simulink model "pendulum_PID"  (R2016a)
settings: Solver=VariableStepAuto  StartTime=0.0  StopTime=50  RelTol=1e-6
values from neighbouring files (symbols this model uses):
  A = [0 1 0 0 ... (first row only)    [main.m]
  B = [0; 1/M; 0; -1/(M*l)]    [main.m]
  C = [1 0 0 0 ... (first row only)    [main.m]
  D = [0; 0; 0; 0]    [main.m]
  K = dlqr(Ad,Bd,Q,R)    [main.m]
  Lwd = Ld(3,:)    [main.m]
  state0 = [x0, dx0, theta0, dtheta0]    [main.m]
undefined symbols (not defined in the file or in its folder): Ad, Bd, Cd, Dd, Den_d, L_db, M_db, Md, Num_d
libraries: simulink x11, fuzblock x2
settings Model: Creator=Maciej  LastModifiedBy=Maciej

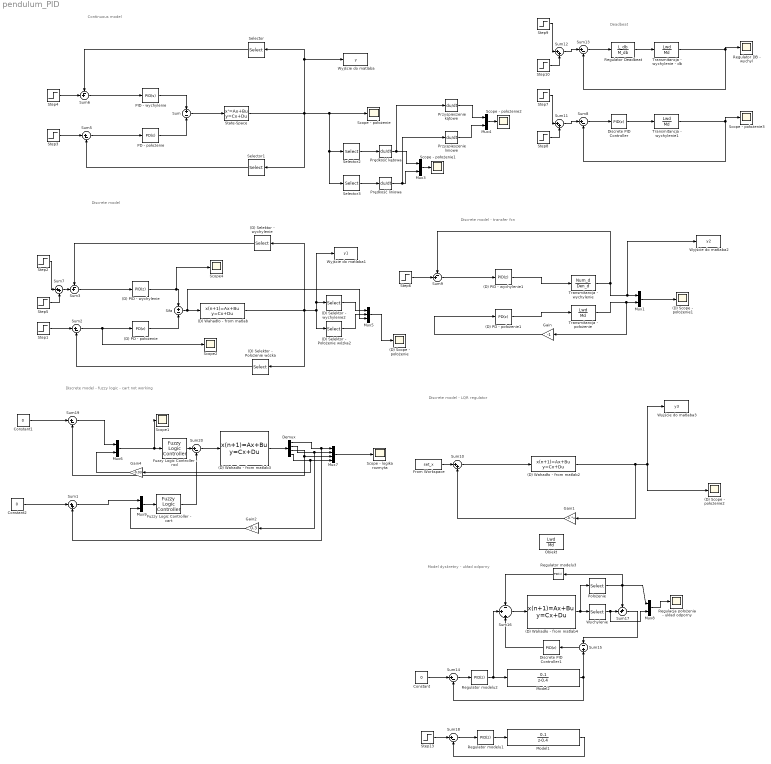
== system pendulum_PID ==
  note: Model dyskretny - układ odporny
  note: Deadbeat
  note: Discrete model - transfer fcn
  note: Discrete model - LQR regulator
  note: Discrete model
  note: Continuous model
  note: Discrete model - fuzzy logic - cart not working
  (D) PD - położenie : simulink/Continuous/PID Controller  Controller=PD  TimeDomain=Discrete-time  SampleTime=0.01  IntegratorMethod=Forward Euler  FilterMethod=Forward Euler  Form=Ideal  UseFilter=off  ControllerParametersSource=internal  P=12.6642993740103  I=0.264679114178146  D=0.005  N=100  InitialConditionSource=internal  InitialConditionForIntegrator=0  InitialConditionForFilter=0  ExternalReset=none  LimitOutput=off  UpperSaturationLimit=inf  LowerSaturationLimit=-inf  LinearizeAsGain=on  AntiWindupMode=none  Kb=1  TrackingMode=off  Kt=1  PParamMin=[]  PParamMax=[]  IParamMin=[]  IParamMax=[]  DParamMin=[]  DParamMax=[]  NParamMin=[]  NParamMax=[]  KbParamMin=[]  KbParamMax=[]  KtParamMin=[]  KtParamMax=[]  POutMin=[]  POutMax=[]  IOutMin=[]  IOutMax=[]  DOutMin=[]  DOutMax=[]  NOutMin=[]  NOutMax=[]  KbOutMin=[]  KbOutMax=[]  KtOutMin=[]  KtOutMax=[]  IntegratorOutMin=[]  IntegratorOutMax=[]  FilterOutMin=[]  FilterOutMax=[]  SumOutMin=[]  SumOutMax=[]  SumI1OutMin=[]  SumI1OutMax=[]  SumI2OutMin=[]  SumI2OutMax=[]  SumI3OutMin=[]  SumI3OutMax=[]  SumDOutMin=[]  SumDOutMax=[]  SaturationOutMin=[]  SaturationOutMax=[]  IntegratorContinuousStateAttributes=''  IntegratorStateMustResolveToSignalObject=off  IntegratorRTWStateStorageClass=Auto  FilterContinuousStateAttributes=''  FilterStateMustResolveToSignalObject=off  FilterRTWStateStorageClass=Auto  DifferentiatorICPrevScaledInput=0  DifferentiatorOutMin=[]  DifferentiatorOutMax=[]
  (D) PD - położenie1 : simulink/Continuous/PID Controller  Controller=PD  TimeDomain=Discrete-time  SampleTime=0.01  IntegratorMethod=Forward Euler  FilterMethod=Trapezoidal  Form=Ideal  UseFilter=on  ControllerParametersSource=internal  P=12.6641410705961  I=0.302421599344656  D=0  N=100  InitialConditionSource=internal  InitialConditionForIntegrator=0  InitialConditionForFilter=0  ExternalReset=none  LimitOutput=off  UpperSaturationLimit=inf  LowerSaturationLimit=-inf  LinearizeAsGain=on  AntiWindupMode=none  Kb=1  TrackingMode=off  Kt=1  PParamMin=[]  PParamMax=[]  IParamMin=[]  IParamMax=[]  DParamMin=[]  DParamMax=[]  NParamMin=[]  NParamMax=[]  KbParamMin=[]  KbParamMax=[]  KtParamMin=[]  KtParamMax=[]  POutMin=[]  POutMax=[]  IOutMin=[]  IOutMax=[]  DOutMin=[]  DOutMax=[]  NOutMin=[]  NOutMax=[]  KbOutMin=[]  KbOutMax=[]  KtOutMin=[]  KtOutMax=[]  IntegratorOutMin=[]  IntegratorOutMax=[]  FilterOutMin=[]  FilterOutMax=[]  SumOutMin=[]  SumOutMax=[]  SumI1OutMin=[]  SumI1OutMax=[]  SumI2OutMin=[]  SumI2OutMax=[]  SumI3OutMin=[]  SumI3OutMax=[]  SumDOutMin=[]  SumDOutMax=[]  SaturationOutMin=[]  SaturationOutMax=[]  IntegratorContinuousStateAttributes=''  IntegratorStateMustResolveToSignalObject=off  IntegratorRTWStateStorageClass=Auto  FilterContinuousStateAttributes=''  FilterStateMustResolveToSignalObject=off  FilterRTWStateStorageClass=Auto  DifferentiatorICPrevScaledInput=0  DifferentiatorOutMin=[]  DifferentiatorOutMax=[]
  (D) PID - wychylenie : simulink/Continuous/PID Controller  Controller=PID  TimeDomain=Discrete-time  SampleTime=0.01  IntegratorMethod=Forward Euler  FilterMethod=Forward Euler  Form=Ideal  UseFilter=on  ControllerParametersSource=internal  P=-46.8558412524277  I=2.71021165385829  D=0.0890699619507767  N=156.758466308077  InitialConditionSource=internal  InitialConditionForIntegrator=0  InitialConditionForFilter=0  ExternalReset=none  LimitOutput=off  UpperSaturationLimit=inf  LowerSaturationLimit=-inf  LinearizeAsGain=on  AntiWindupMode=none  Kb=1  TrackingMode=off  Kt=1  PParamMin=[]  PParamMax=[]  IParamMin=[]  IParamMax=[]  DParamMin=[]  DParamMax=[]  NParamMin=[]  NParamMax=[]  KbParamMin=[]  KbParamMax=[]  KtParamMin=[]  KtParamMax=[]  POutMin=[]  POutMax=[]  IOutMin=[]  IOutMax=[]  DOutMin=[]  DOutMax=[]  NOutMin=[]  NOutMax=[]  KbOutMin=[]  KbOutMax=[]  KtOutMin=[]  KtOutMax=[]  IntegratorOutMin=[]  IntegratorOutMax=[]  FilterOutMin=[]  FilterOutMax=[]  SumOutMin=[]  SumOutMax=[]  SumI1OutMin=[]  SumI1OutMax=[]  SumI2OutMin=[]  SumI2OutMax=[]  SumI3OutMin=[]  SumI3OutMax=[]  SumDOutMin=[]  SumDOutMax=[]  SaturationOutMin=[]  SaturationOutMax=[]  IntegratorContinuousStateAttributes=''  IntegratorStateMustResolveToSignalObject=off  IntegratorRTWStateStorageClass=Auto  FilterContinuousStateAttributes=''  FilterStateMustResolveToSignalObject=off  FilterRTWStateStorageClass=Auto  DifferentiatorICPrevScaledInput=0  DifferentiatorOutMin=[]  DifferentiatorOutMax=[]
  (D) PID - wychylenie1 : simulink/Continuous/PID Controller  Controller=PID  TimeDomain=Discrete-time  SampleTime=0.01  IntegratorMethod=Forward Euler  FilterMethod=Forward Euler  Form=Ideal  UseFilter=on  ControllerParametersSource=internal  P=-46.8558412524277  I=2.71021165385829  D=0.0890699619507767  N=156.758466308077  InitialConditionSource=internal  InitialConditionForIntegrator=0  InitialConditionForFilter=0  ExternalReset=none  LimitOutput=off  UpperSaturationLimit=inf  LowerSaturationLimit=-inf  LinearizeAsGain=on  AntiWindupMode=none  Kb=1  TrackingMode=off  Kt=1  PParamMin=[]  PParamMax=[]  IParamMin=[]  IParamMax=[]  DParamMin=[]  DParamMax=[]  NParamMin=[]  NParamMax=[]  KbParamMin=[]  KbParamMax=[]  KtParamMin=[]  KtParamMax=[]  POutMin=[]  POutMax=[]  IOutMin=[]  IOutMax=[]  DOutMin=[]  DOutMax=[]  NOutMin=[]  NOutMax=[]  KbOutMin=[]  KbOutMax=[]  KtOutMin=[]  KtOutMax=[]  IntegratorOutMin=[]  IntegratorOutMax=[]  FilterOutMin=[]  FilterOutMax=[]  SumOutMin=[]  SumOutMax=[]  SumI1OutMin=[]  SumI1OutMax=[]  SumI2OutMin=[]  SumI2OutMax=[]  SumI3OutMin=[]  SumI3OutMax=[]  SumDOutMin=[]  SumDOutMax=[]  SaturationOutMin=[]  SaturationOutMax=[]  IntegratorContinuousStateAttributes=''  IntegratorStateMustResolveToSignalObject=off  IntegratorRTWStateStorageClass=Auto  FilterContinuousStateAttributes=''  FilterStateMustResolveToSignalObject=off  FilterRTWStateStorageClass=Auto  DifferentiatorICPrevScaledInput=0  DifferentiatorOutMin=[]  DifferentiatorOutMax=[]
  (D) Scope - położenie : Scope
  (D) Scope - położenie1 : Scope
  (D) Scope - położenie2 : Scope
  (D) Selektor - Położenie wózka : Selector  InputPortWidth=4  IndexOptions=Index vector (dialog)  Indices=1  OutputSizes=1
  (D) Selektor - Położenie wózka2 : Selector  InputPortWidth=4  IndexOptions=Index vector (dialog)  Indices=1  OutputSizes=1
  (D) Selektor - wychylenie : Selector  InputPortWidth=4  IndexOptions=Index vector (dialog)  Indices=3  OutputSizes=1
  (D) Selektor - wychylenie2 : Selector  InputPortWidth=4  IndexOptions=Index vector (dialog)  Indices=3  OutputSizes=1
  (D) Wahadło - from matlab{,2..4} (4 alike) : DiscreteStateSpace  A=Ad  B=Bd  C=Cd  D=Dd  X0=state0  SampleTime=0.01
  Constant : Constant  Value=0
  Constant1 : Constant  Value=0  SampleTime=0.01
  Constant2 : Constant  Value=0  SampleTime=0.01
  Demux : Demux
  Discrete PID Controller : simulink/Continuous/PID Controller  Controller=PID  TimeDomain=Discrete-time  SampleTime=0.01  IntegratorMethod=Forward Euler  FilterMethod=Forward Euler  Form=Ideal  UseFilter=off  ControllerParametersSource=internal  P=-50.8  I=7.26  D=0.24  N=100  InitialConditionSource=internal  InitialConditionForIntegrator=0  InitialConditionForFilter=0  ExternalReset=none  LimitOutput=off  UpperSaturationLimit=inf  LowerSaturationLimit=-inf  LinearizeAsGain=off  AntiWindupMode=none  Kb=1  TrackingMode=off  Kt=1  PParamMin=[]  PParamMax=[]  IParamMin=[]  IParamMax=[]  DParamMin=[]  DParamMax=[]  NParamMin=[]  NParamMax=[]  KbParamMin=[]  KbParamMax=[]  KtParamMin=[]  KtParamMax=[]  POutMin=[]  POutMax=[]  IOutMin=[]  IOutMax=[]  DOutMin=[]  DOutMax=[]  NOutMin=[]  NOutMax=[]  KbOutMin=[]  KbOutMax=[]  KtOutMin=[]  KtOutMax=[]  IntegratorOutMin=[]  IntegratorOutMax=[]  FilterOutMin=[]  FilterOutMax=[]  SumOutMin=[]  SumOutMax=[]  SumI1OutMin=[]  SumI1OutMax=[]  SumI2OutMin=[]  SumI2OutMax=[]  SumI3OutMin=[]  SumI3OutMax=[]  SumDOutMin=[]  SumDOutMax=[]  SaturationOutMin=[]  SaturationOutMax=[]  IntegratorContinuousStateAttributes=''  IntegratorStateMustResolveToSignalObject=off  IntegratorRTWStateStorageClass=Auto  FilterContinuousStateAttributes=''  FilterStateMustResolveToSignalObject=off  FilterRTWStateStorageClass=Auto  DifferentiatorICPrevScaledInput=0  DifferentiatorOutMin=[]  DifferentiatorOutMax=[]
  Discrete PID Controller1 : simulink/Continuous/PID Controller  Controller=PID  TimeDomain=Discrete-time  SampleTime=0.01  IntegratorMethod=Forward Euler  FilterMethod=Forward Euler  Form=Ideal  UseFilter=off  ControllerParametersSource=internal  P=-55.2170998286729  I=2.39725052016704  D=0.0822555687688568  N=188.432938311951  InitialConditionSource=internal  InitialConditionForIntegrator=0  InitialConditionForFilter=0  ExternalReset=none  LimitOutput=off  UpperSaturationLimit=inf  LowerSaturationLimit=-inf  LinearizeAsGain=off  AntiWindupMode=none  Kb=1  TrackingMode=off  Kt=1  PParamMin=[]  PParamMax=[]  IParamMin=[]  IParamMax=[]  DParamMin=[]  DParamMax=[]  NParamMin=[]  NParamMax=[]  KbParamMin=[]  KbParamMax=[]  KtParamMin=[]  KtParamMax=[]  POutMin=[]  POutMax=[]  IOutMin=[]  IOutMax=[]  DOutMin=[]  DOutMax=[]  NOutMin=[]  NOutMax=[]  KbOutMin=[]  KbOutMax=[]  KtOutMin=[]  KtOutMax=[]  IntegratorOutMin=[]  IntegratorOutMax=[]  FilterOutMin=[]  FilterOutMax=[]  SumOutMin=[]  SumOutMax=[]  SumI1OutMin=[]  SumI1OutMax=[]  SumI2OutMin=[]  SumI2OutMax=[]  SumI3OutMin=[]  SumI3OutMax=[]  SumDOutMin=[]  SumDOutMax=[]  SaturationOutMin=[]  SaturationOutMax=[]  IntegratorContinuousStateAttributes=''  IntegratorStateMustResolveToSignalObject=off  IntegratorRTWStateStorageClass=Auto  FilterContinuousStateAttributes=''  FilterStateMustResolveToSignalObject=off  FilterRTWStateStorageClass=Auto  DifferentiatorICPrevScaledInput=0  DifferentiatorOutMin=[]  DifferentiatorOutMax=[]
  From Workspace : FromWorkspace  VariableName=set_x  SampleTime=0.01
  Fuzzy Logic Controller - cart : fuzblock/Fuzzy Logic  Controller  fis='regulacja_rozmyta_polozenie.fis'
  Fuzzy Logic Controller - rod : fuzblock/Fuzzy Logic  Controller  fis='regulacja_rozmyta.fis'
  Gain : Gain  Gain=-1
  Gain1 : Gain  Gain=-K  Multiplication=Matrix(K*u)
  Gain2 : Gain  Gain=0.3
  Gain4 : Gain  Gain=-0.03
  Model1 : DiscreteTransferFcn  Numerator=[0.1]  Denominator=[1 -0.4]  SampleTime=0.01
  Model2 : DiscreteTransferFcn  Numerator=[0.1]  Denominator=[1 -0.4]  SampleTime=0.01
  Mux{1,3..4,6,8..9} (6 alike) : Mux  Inputs=2
  Mux5 : Mux  Inputs=3
  Mux7 : Mux
  Obiekt : DiscreteTransferFcn  Numerator=Lwd  Denominator=Md  SampleTime=0.01
  PD - położenie : simulink/Continuous/PID Controller  Controller=PD  TimeDomain=Continuous-time  SampleTime=-1  IntegratorMethod=Forward Euler  FilterMethod=Forward Euler  Form=Ideal  UseFilter=on  ControllerParametersSource=internal  P=12.6641410705961  I=0.302421599344656  D=0  N=100  InitialConditionSource=internal  InitialConditionForIntegrator=0  InitialConditionForFilter=0  ExternalReset=none  LimitOutput=off  UpperSaturationLimit=inf  LowerSaturationLimit=-inf  LinearizeAsGain=on  AntiWindupMode=none  Kb=1  TrackingMode=off  Kt=1  PParamMin=[]  PParamMax=[]  IParamMin=[]  IParamMax=[]  DParamMin=[]  DParamMax=[]  NParamMin=[]  NParamMax=[]  KbParamMin=[]  KbParamMax=[]  KtParamMin=[]  KtParamMax=[]  POutMin=[]  POutMax=[]  IOutMin=[]  IOutMax=[]  DOutMin=[]  DOutMax=[]  NOutMin=[]  NOutMax=[]  KbOutMin=[]  KbOutMax=[]  KtOutMin=[]  KtOutMax=[]  IntegratorOutMin=[]  IntegratorOutMax=[]  FilterOutMin=[]  FilterOutMax=[]  SumOutMin=[]  SumOutMax=[]  SumI1OutMin=[]  SumI1OutMax=[]  SumI2OutMin=[]  SumI2OutMax=[]  SumI3OutMin=[]  SumI3OutMax=[]  SumDOutMin=[]  SumDOutMax=[]  SaturationOutMin=[]  SaturationOutMax=[]  IntegratorContinuousStateAttributes=''  IntegratorStateMustResolveToSignalObject=off  IntegratorRTWStateStorageClass=Auto  FilterContinuousStateAttributes=''  FilterStateMustResolveToSignalObject=off  FilterRTWStateStorageClass=Auto  DifferentiatorICPrevScaledInput=0  DifferentiatorOutMin=[]  DifferentiatorOutMax=[]
  PID - wychylenie : simulink/Continuous/PID Controller  Controller=PID  TimeDomain=Continuous-time  SampleTime=-1  IntegratorMethod=Forward Euler  FilterMethod=Forward Euler  Form=Ideal  UseFilter=on  ControllerParametersSource=internal  P=-46.8558412524277  I=2.71021165385829  D=0.0890699619507767  N=3601.63007352322  InitialConditionSource=internal  InitialConditionForIntegrator=0  InitialConditionForFilter=0  ExternalReset=none  LimitOutput=off  UpperSaturationLimit=inf  LowerSaturationLimit=-inf  LinearizeAsGain=on  AntiWindupMode=none  Kb=1  TrackingMode=off  Kt=1  PParamMin=[]  PParamMax=[]  IParamMin=[]  IParamMax=[]  DParamMin=[]  DParamMax=[]  NParamMin=[]  NParamMax=[]  KbParamMin=[]  KbParamMax=[]  KtParamMin=[]  KtParamMax=[]  POutMin=[]  POutMax=[]  IOutMin=[]  IOutMax=[]  DOutMin=[]  DOutMax=[]  NOutMin=[]  NOutMax=[]  KbOutMin=[]  KbOutMax=[]  KtOutMin=[]  KtOutMax=[]  IntegratorOutMin=[]  IntegratorOutMax=[]  FilterOutMin=[]  FilterOutMax=[]  SumOutMin=[]  SumOutMax=[]  SumI1OutMin=[]  SumI1OutMax=[]  SumI2OutMin=[]  SumI2OutMax=[]  SumI3OutMin=[]  SumI3OutMax=[]  SumDOutMin=[]  SumDOutMax=[]  SaturationOutMin=[]  SaturationOutMax=[]  IntegratorContinuousStateAttributes=''  IntegratorStateMustResolveToSignalObject=off  IntegratorRTWStateStorageClass=Auto  FilterContinuousStateAttributes=''  FilterStateMustResolveToSignalObject=off  FilterRTWStateStorageClass=Auto  DifferentiatorICPrevScaledInput=0  DifferentiatorOutMin=[]  DifferentiatorOutMax=[]
  Położenie : Selector  InputPortWidth=4  IndexOptions=Index vector (dialog)  Indices=1  OutputSizes=1
  Przyspieszenie kątowe : Derivative
  Przyspieszenie liniowe : Derivative
  Prędkość kątowa : Derivative
  Prędkość liniowa : Derivative
  Regulacja położenia - układ odporny : Scope
  Regulator Deadbeat : DiscreteTransferFcn  Numerator=L_db  Denominator=M_db  SampleTime=0.01
  Regulator DB - wychyl : Scope
  Regulator modelu1 : simulink/Continuous/PID Controller  Controller=PID  TimeDomain=Discrete-time  SampleTime=0.01  IntegratorMethod=Forward Euler  FilterMethod=Forward Euler  Form=Ideal  UseFilter=off  ControllerParametersSource=internal  P=1.93752687309823  I=100  D=0.0025  N=100  InitialConditionSource=internal  InitialConditionForIntegrator=0  InitialConditionForFilter=0  ExternalReset=none  LimitOutput=off  UpperSaturationLimit=inf  LowerSaturationLimit=-inf  LinearizeAsGain=off  AntiWindupMode=none  Kb=1  TrackingMode=off  Kt=1  PParamMin=[]  PParamMax=[]  IParamMin=[]  IParamMax=[]  DParamMin=[]  DParamMax=[]  NParamMin=[]  NParamMax=[]  KbParamMin=[]  KbParamMax=[]  KtParamMin=[]  KtParamMax=[]  POutMin=[]  POutMax=[]  IOutMin=[]  IOutMax=[]  DOutMin=[]  DOutMax=[]  NOutMin=[]  NOutMax=[]  KbOutMin=[]  KbOutMax=[]  KtOutMin=[]  KtOutMax=[]  IntegratorOutMin=[]  IntegratorOutMax=[]  FilterOutMin=[]  FilterOutMax=[]  SumOutMin=[]  SumOutMax=[]  SumI1OutMin=[]  SumI1OutMax=[]  SumI2OutMin=[]  SumI2OutMax=[]  SumI3OutMin=[]  SumI3OutMax=[]  SumDOutMin=[]  SumDOutMax=[]  SaturationOutMin=[]  SaturationOutMax=[]  IntegratorContinuousStateAttributes=''  IntegratorStateMustResolveToSignalObject=off  IntegratorRTWStateStorageClass=Auto  FilterContinuousStateAttributes=''  FilterStateMustResolveToSignalObject=off  FilterRTWStateStorageClass=Auto  DifferentiatorICPrevScaledInput=0  DifferentiatorOutMin=[]  DifferentiatorOutMax=[]
  Regulator modelu2 : simulink/Continuous/PID Controller  Controller=PID  TimeDomain=Discrete-time  SampleTime=0.01  IntegratorMethod=Forward Euler  FilterMethod=Forward Euler  Form=Ideal  UseFilter=off  ControllerParametersSource=internal  P=1.93752687309823  I=100  D=0.0025  N=100  InitialConditionSource=internal  InitialConditionForIntegrator=0  InitialConditionForFilter=0  ExternalReset=none  LimitOutput=off  UpperSaturationLimit=inf  LowerSaturationLimit=-inf  LinearizeAsGain=off  AntiWindupMode=none  Kb=1  TrackingMode=off  Kt=1  PParamMin=[]  PParamMax=[]  IParamMin=[]  IParamMax=[]  DParamMin=[]  DParamMax=[]  NParamMin=[]  NParamMax=[]  KbParamMin=[]  KbParamMax=[]  KtParamMin=[]  KtParamMax=[]  POutMin=[]  POutMax=[]  IOutMin=[]  IOutMax=[]  DOutMin=[]  DOutMax=[]  NOutMin=[]  NOutMax=[]  KbOutMin=[]  KbOutMax=[]  KtOutMin=[]  KtOutMax=[]  IntegratorOutMin=[]  IntegratorOutMax=[]  FilterOutMin=[]  FilterOutMax=[]  SumOutMin=[]  SumOutMax=[]  SumI1OutMin=[]  SumI1OutMax=[]  SumI2OutMin=[]  SumI2OutMax=[]  SumI3OutMin=[]  SumI3OutMax=[]  SumDOutMin=[]  SumDOutMax=[]  SaturationOutMin=[]  SaturationOutMax=[]  IntegratorContinuousStateAttributes=''  IntegratorStateMustResolveToSignalObject=off  IntegratorRTWStateStorageClass=Auto  FilterContinuousStateAttributes=''  FilterStateMustResolveToSignalObject=off  FilterRTWStateStorageClass=Auto  DifferentiatorICPrevScaledInput=0  DifferentiatorOutMin=[]  DifferentiatorOutMax=[]
  Regulator modelu3 : simulink/Continuous/PID Controller  Controller=PID  TimeDomain=Discrete-time  SampleTime=0.01  IntegratorMethod=Forward Euler  FilterMethod=Forward Euler  Form=Ideal  UseFilter=off  ControllerParametersSource=internal  P=-18.1852230940277  I=1.21597236750382  D=0.205596777263215  N=100  InitialConditionSource=internal  InitialConditionForIntegrator=0  InitialConditionForFilter=0  ExternalReset=none  LimitOutput=off  UpperSaturationLimit=inf  LowerSaturationLimit=-inf  LinearizeAsGain=off  AntiWindupMode=none  Kb=1  TrackingMode=off  Kt=1  PParamMin=[]  PParamMax=[]  IParamMin=[]  IParamMax=[]  DParamMin=[]  DParamMax=[]  NParamMin=[]  NParamMax=[]  KbParamMin=[]  KbParamMax=[]  KtParamMin=[]  KtParamMax=[]  POutMin=[]  POutMax=[]  IOutMin=[]  IOutMax=[]  DOutMin=[]  DOutMax=[]  NOutMin=[]  NOutMax=[]  KbOutMin=[]  KbOutMax=[]  KtOutMin=[]  KtOutMax=[]  IntegratorOutMin=[]  IntegratorOutMax=[]  FilterOutMin=[]  FilterOutMax=[]  SumOutMin=[]  SumOutMax=[]  SumI1OutMin=[]  SumI1OutMax=[]  SumI2OutMin=[]  SumI2OutMax=[]  SumI3OutMin=[]  SumI3OutMax=[]  SumDOutMin=[]  SumDOutMax=[]  SaturationOutMin=[]  SaturationOutMax=[]  IntegratorContinuousStateAttributes=''  IntegratorStateMustResolveToSignalObject=off  IntegratorRTWStateStorageClass=Auto  FilterContinuousStateAttributes=''  FilterStateMustResolveToSignalObject=off  FilterRTWStateStorageClass=Auto  DifferentiatorICPrevScaledInput=0  DifferentiatorOutMin=[]  DifferentiatorOutMax=[]
  Scope - logika rozmyta : Scope
  Scope - położenie{,1..3} (4 alike) : Scope
  Scope1 : Scope
  Scope2 : Scope
  Scope4 : Scope
  Selector : Selector  InputPortWidth=4  IndexOptions=Index vector (dialog)  Indices=3  OutputSizes=1
  Selector1 : Selector  InputPortWidth=4  IndexOptions=Index vector (dialog)  Indices=1  OutputSizes=1
  Selector2 : Selector  InputPortWidth=4  IndexOptions=Index vector (dialog)  Indices=3  OutputSizes=1
  Selector3 : Selector  InputPortWidth=4  IndexOptions=Index vector (dialog)  Indices=1  OutputSizes=1
  Siła : Sum  Inputs=+|-
  State-Space : StateSpace  A=A  B=B  C=C  D=D  X0=state0
  Step1 : Step  Time=0  After=0  SampleTime=0.01
  Step10 : Step  Time=0  After=pi/10  SampleTime=0.01
  Step13 : Step  Time=0  After=pi/10  SampleTime=0.01
  Step2 : Step  After=0  SampleTime=0
  Step3 : Step  Time=0  After=0  SampleTime=0
  Step4 : Step  Time=0  After=0  SampleTime=0
  Step5 : Step  Time=0  After=0  SampleTime=0
  Step6 : Step  After=0  SampleTime=0.01
  Step7 : Step  Time=0  Before=pi/10  After=0  SampleTime=0.01
  Step8 : Step  Time=0  After=pi/10  SampleTime=0.01
  Step9 : Step  Time=0  Before=pi/10  After=0  SampleTime=0.01
  Sum : Sum  Inputs=+-
  Sum{1,7,10..12} (5 alike) : Sum  Inputs=|++
  Sum{2,5,8,13..14,18..20} (8 alike) : Sum  Inputs=|+-
  Sum15 : Sum  Inputs=-|+
  Sum16 : Sum  Inputs=-|+|+
  Sum17 : Sum  Inputs=++|
  Sum3 : Sum  Inputs=-+|
  Sum6 : Sum  Inputs=-+|
  Sum9 : Sum  Inputs=-+|
  Transmitancja - położenie : DiscreteTransferFcn  Numerator=Lwd  Denominator=Md  SampleTime=0.01
  Transmitancja - wychylenie : DiscreteTransferFcn  Numerator=Num_d  Denominator=Den_d  InitialStates=0.316  SampleTime=0.01
  Transmitancja - wychylenie - db : DiscreteTransferFcn  Numerator=Lwd  Denominator=Md  SampleTime=0.01
  Transmitancja - wychylenie1 : DiscreteTransferFcn  Numerator=Lwd  Denominator=Md  SampleTime=0.01
  Wychylenie : Selector  InputPortWidth=4  IndexOptions=Index vector (dialog)  Indices=3  OutputSizes=1
  Wyjście do matlaba : ToWorkspace  VariableName=y  SampleTime=-1
  Wyjście do matlaba1 : ToWorkspace  VariableName=y1  SampleTime=-1
  Wyjście do matlaba2 : ToWorkspace  VariableName=y2  SampleTime=-1
  Wyjście do matlaba3 : ToWorkspace  VariableName=y3  SampleTime=-1
  wires:
  PD - położenie/1 -> Sum/2
  Step3/1 -> Sum5/1
  Sum5/1 -> PD - położenie/1
  Step4/1 -> Sum6/2
  Sum6/1 -> PID - wychylenie/1
  State-Space/1 -> Selector1/1, Selector3/1, Selector2/1, Scope - położenie/1, Selector/1, Wyjście do matlaba/1
  (D) PID - wychylenie/1 -> Scope4/1, Siła/1
  (D) PD - położenie/1 -> Siła/2
  Siła/1 -> Mux5/3, (D) Wahadło - from matlab/1
  Step1/1 -> Sum2/1
  Sum2/1 -> Scope2/1, (D) PD - położenie/1
  Sum3/1 -> (D) PID - wychylenie/1
  (D) Wahadło - from matlab/1 -> (D) Selektor - Położenie wózka/1, (D) Selektor - wychylenie2/1, Wyjście do matlaba1/1, (D) Selektor - Położenie wózka2/1, (D) Selektor - wychylenie/1
  (D) Selektor - Położenie wózka/1 -> Sum2/2
  (D) Selektor - wychylenie/1 -> Sum3/1
  (D) PID - wychylenie1/1 -> Transmitancja - wychylenie/1
  (D) PD - położenie1/1 -> Transmitancja - położenie/1
  Transmitancja - położenie/1 -> Gain/1, Mux1/2
  Step6/1 -> Sum9/2
  Sum9/1 -> (D) PID - wychylenie1/1
  Mux1/1 -> (D) Scope - położenie1/1
  Selector/1 -> Sum6/1
  Selector1/1 -> Sum5/2
  Sum/1 -> State-Space/1
  PID - wychylenie/1 -> Sum/1
  Transmitancja - wychylenie/1 -> Sum9/1, Wyjście do matlaba2/1, Mux1/1
  (D) Wahadło - from matlab2/1 -> Gain1/1, (D) Scope - położenie2/1, Wyjście do matlaba3/1
  Gain1/1 -> Sum10/2
  Sum10/1 -> (D) Wahadło - from matlab2/1
  From Workspace/1 -> Sum10/1
  Selector3/1 -> Prędkość liniowa/1
  Selector2/1 -> Prędkość kątowa/1
  Mux3/1 -> Scope - położenie1/1
  Prędkość liniowa/1 -> Przyspieszenie liniowe/1, Mux3/2
  Prędkość kątowa/1 -> Przyspieszenie kątowe/1, Mux3/1
  Przyspieszenie liniowe/1 -> Mux4/2
  Przyspieszenie kątowe/1 -> Mux4/1
  Mux4/1 -> Scope - położenie2/1
  (D) Selektor - Położenie wózka2/1 -> Mux5/2
  (D) Selektor - wychylenie2/1 -> Mux5/1
  Mux5/1 -> (D) Scope - położenie/1
  Discrete PID Controller/1 -> Transmitancja - wychylenie1/1
  Sum8/1 -> Discrete PID Controller/1
  Transmitancja - wychylenie1/1 -> Sum8/2, Scope - położenie3/1
  (D) Wahadło - from matlab3/1 -> Demux/1
  Mux7/1 -> Scope - logika rozmyta/1
  Gain/1 -> (D) PD - położenie1/1
  Sum7/1 -> Sum3/2
  Step2/1 -> Sum7/1
  Step5/1 -> Sum7/2
  Step8/1 -> Sum11/2
  Sum11/1 -> Sum8/1
  Step7/1 -> Sum11/1
  Sum13/1 -> Regulator Deadbeat/1
  Transmitancja - wychylenie - db/1 -> Regulator DB - wychyl/1, Sum13/2
  Step10/1 -> Sum12/2
  Sum12/1 -> Sum13/1
  Step9/1 -> Sum12/1
  Regulator Deadbeat/1 -> Transmitancja - wychylenie - db/1
  Sum14/1 -> Regulator modelu2/1
  Regulator modelu2/1 -> Model2/1, Sum16/2
  Model2/1 -> Sum15/2, Sum14/2
  Sum15/1 -> Discrete PID Controller1/1
  Discrete PID Controller1/1 -> Sum16/3
  Constant/1 -> Sum14/1
  Regulator modelu1/1 -> Model1/1
  Sum18/1 -> Regulator modelu1/1
  Step13/1 -> Sum18/1
  Model1/1 -> Sum18/2
  Sum16/1 -> (D) Wahadło - from matlab4/1
  Sum17/1 -> Sum15/1
  Wychylenie/1 -> Mux8/2, Sum17/2
  Położenie/1 -> Sum17/1, Regulator modelu3/1, Mux8/1
  Mux8/1 -> Regulacja położenia - układ odporny/1
  (D) Wahadło - from matlab4/1 -> Położenie/1, Wychylenie/1
  Demux/3 -> Sum19/2, Mux7/3
  Sum19/1 -> Mux6/1
  Constant1/1 -> Sum19/1
  Mux6/1 -> Scope1/1, Fuzzy Logic Controller - rod/1
  Fuzzy Logic Controller - rod/1 -> Sum20/1
  Regulator modelu3/1 -> Sum16/1
  Constant2/1 -> Sum1/1
  Demux/1 -> Sum1/2, Mux7/1
  Demux/2 -> Gain2/1, Mux7/2
  Demux/4 -> Gain4/1, Mux7/4
  Mux9/1 -> Fuzzy Logic Controller - cart/1
  Gain4/1 -> Mux6/2
  Gain2/1 -> Mux9/2
  Fuzzy Logic Controller - cart/1 -> Sum20/2
  Sum1/1 -> Mux9/1
  Sum20/1 -> (D) Wahadło - from matlab3/1
